simulink model "TeamA_PAsqualo1"  (R2020a)
settings: Solver=VariableStepAuto  StartTime=0.0  StopTime=stop_time  FixedStep=0.05  RelTol=1e-3
InitFcn:
  | main_init
values from neighbouring files (symbols this model uses):
  a1 = rho * D^4 * alpha1    (= 0.000388302366464)    [data_current.m]    (also in main_init.m)
  a2 = -rho * D^3 * alpha2 * (1 - omega)    (= 0.0037030698432)    [data_current.m]    (also in main_init.m)
  ag = [Ax Ay Az]'    [init_modello.m]
  alpha1 = 0.0113    [data_current.m]    (also in main_init.m)
  alpha2 = -0.0091    [data_current.m]    (also in main_init.m)
  areaOfInterestCorner = [42.317744;10.915136; 0]    [init_controllo.m]    (also in missionA.m = [42.317744)
  bg = [Bx By Bz]'    [init_modello.m]
  cd_pitch = 0.7    [init_modello.m]
  cd_roll = 0.04    [init_modello.m]
  cd_x = 0.4    [init_modello.m]
  cd_y = 1    [init_modello.m]
  cd_yaw = 0.7    [init_modello.m]
  cd_z = 1    [init_modello.m]
  cg = [Cx Cy Cz]'    [init_modello.m]
  D = 0.076    [data_current.m]    (also in main_init.m)
  dead_zone_limit = 31.5    [data_current.m]    (also in main_init.m)
  dg = [Dx Dy Dz]'    [init_modello.m]
  eg = [Ex Ey Ez]'    [init_modello.m]
  fg = [Fx Fy Fz]'    [init_modello.m]
  g = 9.81    [init_modello.m]
  galleggiamento = 66.5386    [init_controllo.m]
  gg = [Gx Gy Gz]'    [init_modello.m]
  H0 = 0    [init_modello.m]
  init_position = [pointP(1),pointP(2),0.15,0,0,deg2rad(angle)]'    [appunti.m]    (also in init_modello.m = [pointP(1),pointP(2),0.15,0,0,deg2rad(alpha)]')
  init_velocity = [0 0 0 0 0 0]'    [init_modello.m]
  initial_state_cov = blkdiag(diag(cov_gps(1,1:2)), cov_depth*eye(n_state_filter-2))    [init_navigazione.m]
  Ixx = 0.93304097392    [init_modello.m]
  Ixy = 0    [init_modello.m]
  Ixz = 0    [init_modello.m]
  Iyy = 25.58745481378    (= 25.5874548138)    [init_modello.m]
  Iyz = 0    [init_modello.m]
  Izz = 25.58745481378    (= 25.5874548138)    [init_modello.m]
  K_i_heave_div = 20    [init_controllo.m]
  K_i_heave_pos = 1    [init_controllo.m]
  K_i_heave_surf = 20    [init_controllo.m]
  K_i_heave_trans = 5    [init_controllo.m]
  K_i_heave_turn = 5    [init_controllo.m]
  K_i_pitch_div = 0    [init_controllo.m]
  K_i_pitch_pos = 0.1*0    (= 0)    [init_controllo.m]
  K_i_pitch_surf = 0    [init_controllo.m]
  K_i_pitch_trans = 0    [init_controllo.m]
  K_i_pitch_turn = 0    [init_controllo.m]
  K_i_roll_div = 0    [init_controllo.m]
  K_i_roll_pos = 0.1*0    (= 0)    [init_controllo.m]
  K_i_roll_surf = 1    [init_controllo.m]
  K_i_roll_trans = 0    [init_controllo.m]
  K_i_roll_turn = 0    [init_controllo.m]
  K_i_surge_div = 3    [init_controllo.m]
  K_i_surge_pos = 0.1679*30    (= 5.037)    [init_controllo.m]
  K_i_surge_surf = 3    [init_controllo.m]
  K_i_surge_trans = 0.1679*15    (= 2.5185)    [init_controllo.m]
  K_i_surge_turn = 0.1679*60    (= 10.074)    [init_controllo.m]
  K_i_sway_div = 6    [init_controllo.m]
  K_i_sway_pos = 5    [init_controllo.m]
  K_i_sway_surf = 3    [init_controllo.m]
  K_i_sway_trans = 2    [init_controllo.m]
  K_i_sway_turn = 50    [init_controllo.m]
  K_i_yaw_div = 0    [init_controllo.m]
  K_i_yaw_pos = 1    [init_controllo.m]
  K_i_yaw_surf = 0    [init_controllo.m]
  K_i_yaw_trans = 20    [init_controllo.m]
  K_i_yaw_turn = 3    [init_controllo.m]
  K_p_heave_div = 200    [init_controllo.m]
  K_p_heave_pos = 320    [init_controllo.m]
  K_p_heave_surf = 200    [init_controllo.m]
  K_p_heave_trans = 170    [init_controllo.m]
  K_p_heave_turn = 170    [init_controllo.m]
  K_p_phi_div = 0.15    [init_controllo.m]
  K_p_phi_pos = 1*0.1    (= 0.1)    [init_controllo.m]
  K_p_phi_surf = 0.15    [init_controllo.m]
  K_p_phi_trans = 0.1    [init_controllo.m]
  K_p_phi_turn = 0.1    [init_controllo.m]
  K_p_pitch_div = 50    [init_controllo.m]
  K_p_pitch_pos = 25    [init_controllo.m]
  K_p_pitch_surf = 50    [init_controllo.m]
  K_p_pitch_trans = 25    [init_controllo.m]
  K_p_pitch_turn = 25    [init_controllo.m]
  K_p_psi_div = 0.3    [init_controllo.m]
  K_p_psi_pos = 0.25    [init_controllo.m]
  K_p_psi_surf = 0.3    [init_controllo.m]
  K_p_psi_trans = 0.2    [init_controllo.m]
  K_p_roll_div = 10    [init_controllo.m]
  K_p_roll_pos = 0.1*40    (= 4)    [init_controllo.m]
  K_p_roll_surf = 10    [init_controllo.m]
  K_p_roll_trans = 0.1*40    (= 4)    [init_controllo.m]
  K_p_roll_turn = 4    [init_controllo.m]
  K_p_surge_div = 80    [init_controllo.m]
  K_p_surge_pos = 13.7782*2.5    (= 34.4455)    [init_controllo.m]
  K_p_surge_surf = 80    [init_controllo.m]
  K_p_surge_trans = 20    [init_controllo.m]
  K_p_surge_turn = 150    [init_controllo.m]
  K_p_sway_div = 100    [init_controllo.m]
  K_p_sway_pos = 90    [init_controllo.m]
  K_p_sway_surf = 80    [init_controllo.m]
  K_p_sway_trans = 80    [init_controllo.m]
  K_p_sway_turn = 200    [init_controllo.m]
  K_p_th_div = 0.3    [init_controllo.m]
  K_p_th_pos = 0.1    [init_controllo.m]
  K_p_th_surf = 0.3    [init_controllo.m]
  K_p_th_trans = 0.1    [init_controllo.m]
  K_p_th_turn = 0.1    [init_controllo.m]
  K_p_x_div = 0.12    [init_controllo.m]
  K_p_x_pos = 0.12    [init_controllo.m]
  K_p_x_surf = 0.12    [init_controllo.m]
  K_p_y_div = 0.6    [init_controllo.m]
  K_p_y_pos = 0.34    [init_controllo.m]
  K_p_y_surf = 0.1    [init_controllo.m]
  K_p_y_trans = 0.3    [init_controllo.m]
  K_p_y_turn = 0.3    [init_controllo.m]
  K_p_yaw_div = 70    [init_controllo.m]
  K_p_yaw_pos = 20    [init_controllo.m]
  K_p_yaw_surf = 70    [init_controllo.m]
  K_p_yaw_trans = 160    [init_controllo.m]
  K_p_yaw_turn = 60    [init_controllo.m]
  K_p_z_div = 0.35    [init_controllo.m]
  K_p_z_pos = 0.2    [init_controllo.m]
  K_p_z_surf = 0.35    [init_controllo.m]
  K_p_z_trans = 0.10    (= 0.1)    [init_controllo.m]
  K_p_z_turn = 0.1    [init_controllo.m]
  Kadd = 0    [init_modello.m]
  ... (+61 more)
undefined symbols (not defined in the file or in its folder): DiscIntNeverNeededParam, initial_state
libraries: simulink x4, vrlib x1
(part 3 of 6)

== system TeamA_PAsqualo1/Controller/surfacing controller/pitch_controller/Pitch PID controller ==
  enable : Inport
  references : Inport  Port=2
  "estimated measures " : Inport  Port=3
  Constant : Constant
  Constant1 : Constant  Value=0
  Discrete-Time Integrator : DiscreteIntegrator  ExternalReset=falling  SampleTime=0.1  ICPrevOutput=DiscIntNeverNeededParam  ICPrevScaledInput=DiscIntNeverNeededParam
  K_i_pitch_surf : Gain  Gain=K_i_pitch_surf
  K_p_pitch_surf : Gain  Gain=K_p_pitch_surf
  K_p_th_surf : Gain  Gain=K_p_th_surf
  Sum2 : Sum
  Switch : Switch  Threshold=1
  compute_orientation_errors : MATLAB Function  TreatAsAtomicUnit=on
  compute_velocity_error : MATLAB Function  TreatAsAtomicUnit=on
  M : Outport
  wires:
  references/1 -> compute_orientation_errors/2(ref)
  K_p_th_surf/1 -> compute_velocity_error/2(v_des)
  "estimated measures "/1 -> compute_velocity_error/3(est_meas), compute_orientation_errors/3(est_state)
  compute_orientation_errors/1(err_orient) -> K_p_th_surf/1  "err_orient"
  Sum2/1 -> M/1
  Discrete-Time Integrator/1 -> Sum2/2
  K_i_pitch_surf/1 -> Discrete-Time Integrator/1
  K_p_pitch_surf/1 -> Sum2/1
  compute_velocity_error/1(err_vel) -> K_i_pitch_surf/1, K_p_pitch_surf/1  "err_vel"
  Switch/1 -> Discrete-Time Integrator/2
  enable/1 -> Switch/2, compute_velocity_error/1(enable), compute_orientation_errors/1(enable)
  Constant1/1 -> Switch/3
  Constant/1 -> Switch/1

== system TeamA_PAsqualo1/Controller/surfacing controller/roll_controller/Roll PID controller ==
  enable : Inport
  references : Inport  Port=2
  "estimated measures " : Inport  Port=3
  Constant : Constant
  Constant1 : Constant  Value=0
  Discrete-Time Integrator : DiscreteIntegrator  ExternalReset=falling  SampleTime=0.1  ICPrevOutput=DiscIntNeverNeededParam  ICPrevScaledInput=DiscIntNeverNeededParam
  K_i_roll_surf : Gain  Gain=K_i_roll_surf
  K_p_phi_surf : Gain  Gain=K_p_phi_surf
  K_p_roll_surf : Gain  Gain=K_p_roll_surf
  Sum2 : Sum
  Switch : Switch  Threshold=1
  compute_orientation_errors : MATLAB Function  TreatAsAtomicUnit=on
  compute_velocity_error : MATLAB Function  TreatAsAtomicUnit=on
  K : Outport
  wires:
  "estimated measures "/1 -> compute_velocity_error/3(est_meas), compute_orientation_errors/3(est_state)
  K_p_phi_surf/1 -> compute_velocity_error/2(v_des)
  compute_orientation_errors/1(err_orient) -> K_p_phi_surf/1  "err_orient"
  references/1 -> compute_orientation_errors/2(ref)
  Sum2/1 -> K/1
  Discrete-Time Integrator/1 -> Sum2/2
  K_i_roll_surf/1 -> Discrete-Time Integrator/1
  K_p_roll_surf/1 -> Sum2/1
  compute_velocity_error/1(err_vel) -> K_i_roll_surf/1, K_p_roll_surf/1  "err_vel"
  Switch/1 -> Discrete-Time Integrator/2
  enable/1 -> Switch/2, compute_velocity_error/1(enable), compute_orientation_errors/1(enable)
  Constant1/1 -> Switch/3
  Constant/1 -> Switch/1

== system TeamA_PAsqualo1/Controller/surfacing controller/surge_controller/Surge PID controller ==
  enable : Inport
  references : Inport  Port=2
  "estimated measures " : Inport  Port=3
  Constant : Constant
  Constant1 : Constant  Value=0
  Discrete-Time Integrator : DiscreteIntegrator  ExternalReset=falling  SampleTime=0.1  ICPrevOutput=DiscIntNeverNeededParam  ICPrevScaledInput=DiscIntNeverNeededParam
  K_i_surge_surf : Gain  Gain=K_i_surge_surf
  K_p_surge_surf : Gain  Gain=K_p_surge_surf
  K_p_x_surf : Gain  Gain=K_p_x_surf
  Sum2 : Sum
  Switch : Switch  Threshold=1
  compute_position_errors : MATLAB Function  TreatAsAtomicUnit=on
  compute_velocity_error : MATLAB Function  TreatAsAtomicUnit=on
  X : Outport
  wires:
  references/1 -> compute_position_errors/2(ref)
  compute_position_errors/1(err_pos) -> K_p_x_surf/1  "err_vect"
  K_p_x_surf/1 -> compute_velocity_error/2(v_des)
  "estimated measures "/1 -> compute_velocity_error/3(est_meas), compute_position_errors/3(est_state)
  K_i_surge_surf/1 -> Discrete-Time Integrator/1
  K_p_surge_surf/1 -> Sum2/1
  Sum2/1 -> X/1
  compute_velocity_error/1(err_vel) -> K_i_surge_surf/1, K_p_surge_surf/1  "err_vel"
  Discrete-Time Integrator/1 -> Sum2/2
  Switch/1 -> Discrete-Time Integrator/2
  enable/1 -> Switch/2, compute_velocity_error/1(enable), compute_position_errors/1(enable)
  Constant1/1 -> Switch/3
  Constant/1 -> Switch/1

== system TeamA_PAsqualo1/Controller/surfacing controller/sway_controller/Sway PID controller ==
  enable : Inport
  references : Inport  Port=2
  "estimated measures " : Inport  Port=3
  Constant : Constant
  Constant1 : Constant  Value=0
  Discrete-Time Integrator : DiscreteIntegrator  ExternalReset=falling  SampleTime=0.1  ICPrevOutput=DiscIntNeverNeededParam  ICPrevScaledInput=DiscIntNeverNeededParam
  K_i_sway_surf : Gain  Gain=K_i_sway_surf
  K_p_sway_surf : Gain  Gain=K_p_sway_surf
  K_p_y_surf : Gain  Gain=K_p_y_surf
  Sum2 : Sum
  Switch : Switch  Threshold=1
  compute_position_errors : MATLAB Function  TreatAsAtomicUnit=on
  compute_velocity_error : MATLAB Function  TreatAsAtomicUnit=on
  Y : Outport
  wires:
  references/1 -> compute_position_errors/2(ref)
  compute_position_errors/1(err_pos) -> K_p_y_surf/1  "err_y"
  K_p_y_surf/1 -> compute_velocity_error/2(v_des)
  "estimated measures "/1 -> compute_velocity_error/3(est_meas), compute_position_errors/3(est_state)
  K_i_sway_surf/1 -> Discrete-Time Integrator/1
  K_p_sway_surf/1 -> Sum2/1
  Sum2/1 -> Y/1
  compute_velocity_error/1(err_vel) -> K_i_sway_surf/1, K_p_sway_surf/1  "err_vel"
  Discrete-Time Integrator/1 -> Sum2/2
  Switch/1 -> Discrete-Time Integrator/2
  enable/1 -> Switch/2, compute_velocity_error/1(enable), compute_position_errors/1(enable)
  Constant1/1 -> Switch/3
  Constant/1 -> Switch/1

== system TeamA_PAsqualo1/Controller/surfacing controller/yaw_controller/Yaw PID controller ==
  enable : Inport
  references : Inport  Port=2
  "estimated measures " : Inport  Port=3
  Constant : Constant
  Constant1 : Constant  Value=0
  Discrete-Time Integrator : DiscreteIntegrator  ExternalReset=falling  SampleTime=0.1  ICPrevOutput=DiscIntNeverNeededParam  ICPrevScaledInput=DiscIntNeverNeededParam
  K_i_yaw_surf : Gain  Gain=K_i_yaw_surf
  K_p_psi_surf : Gain  Gain=K_p_psi_surf
  K_p_yaw_surf : Gain  Gain=K_p_yaw_surf
  Sum2 : Sum
  Switch : Switch  Threshold=1
  compute_orientation_errors : MATLAB Function  TreatAsAtomicUnit=on
  compute_velocity_error : MATLAB Function  TreatAsAtomicUnit=on
  N : Outport
  wires:
  references/1 -> compute_orientation_errors/2(ref)
  "estimated measures "/1 -> compute_velocity_error/3(est_meas), compute_orientation_errors/3(est_state)
  compute_orientation_errors/1(err_orient) -> K_p_psi_surf/1  "err_orient"
  K_p_psi_surf/1 -> compute_velocity_error/2(v_des)
  Sum2/1 -> N/1
  Discrete-Time Integrator/1 -> Sum2/2
  K_i_yaw_surf/1 -> Discrete-Time Integrator/1
  K_p_yaw_surf/1 -> Sum2/1
  compute_velocity_error/1(err_vel) -> K_i_yaw_surf/1, K_p_yaw_surf/1  "err_vel"
  Switch/1 -> Discrete-Time Integrator/2
  enable/1 -> Switch/2, compute_velocity_error/1(enable), compute_orientation_errors/1(enable)
  Constant1/1 -> Switch/3
  Constant/1 -> Switch/1

== system TeamA_PAsqualo1/Controller/transect controller/heave_controller/Heave PID controller ==
  enable : Inport
  references : Inport  Port=2
  "estimated measures " : Inport  Port=3
  Constant : Constant  Value=galleggiamento
  Constant1 : Constant
  Constant2 : Constant  Value=0
  Discrete-Time Integrator : DiscreteIntegrator  ExternalReset=falling  InitialConditionSource=external  SampleTime=0.1  ICPrevOutput=DiscIntNeverNeededParam  ICPrevScaledInput=DiscIntNeverNeededParam
  K_i_heave_trans : Gain  Gain=K_i_heave_trans
  K_p_heave_trans : Gain  Gain=K_p_heave_trans
  K_p_z_trans : Gain  Gain=K_p_z_trans
  Sum2 : Sum
  Switch : Switch  Threshold=1
  compute_position_errors : MATLAB Function  TreatAsAtomicUnit=on
  compute_velocity_error : MATLAB Function  TreatAsAtomicUnit=on
  Z : Outport
  wires:
  "estimated measures "/1 -> compute_velocity_error/3(est_meas), compute_position_errors/3(est_state)
  K_p_z_trans/1 -> compute_velocity_error/2(v_des)
  compute_position_errors/1(err_pos) -> K_p_z_trans/1  "err_vect"
  references/1 -> compute_position_errors/2(ref)
  Sum2/1 -> Z/1
  Discrete-Time Integrator/1 -> Sum2/2
  K_p_heave_trans/1 -> Sum2/1
  K_i_heave_trans/1 -> Discrete-Time Integrator/1
  compute_velocity_error/1(err_vel) -> K_i_heave_trans/1, K_p_heave_trans/1  "err_vel"
  Constant/1 -> Discrete-Time Integrator/3
  Switch/1 -> Discrete-Time Integrator/2
  enable/1 -> Switch/2, compute_velocity_error/1(enable), compute_position_errors/1(enable)
  Constant2/1 -> Switch/3
  Constant1/1 -> Switch/1

== system TeamA_PAsqualo1/Controller/transect controller/pitch_controller/Pitch PID controller ==
  enable : Inport
  references : Inport  Port=2
  "estimated measures " : Inport  Port=3
  Constant : Constant
  Constant1 : Constant  Value=0
  Discrete-Time Integrator : DiscreteIntegrator  ExternalReset=falling  SampleTime=0.1  ICPrevOutput=DiscIntNeverNeededParam  ICPrevScaledInput=DiscIntNeverNeededParam
  K_i_pitch_trans : Gain  Gain=K_i_pitch_trans
  K_p_pitch_trans : Gain  Gain=K_p_pitch_trans
  K_p_th_trans : Gain  Gain=K_p_th_trans
  Sum2 : Sum
  Switch : Switch  Threshold=1
  compute_orientation_errors : MATLAB Function  TreatAsAtomicUnit=on
  compute_velocity_error : MATLAB Function  TreatAsAtomicUnit=on
  M : Outport
  wires:
  references/1 -> compute_orientation_errors/2(ref)
  K_p_th_trans/1 -> compute_velocity_error/2(v_des)
  "estimated measures "/1 -> compute_velocity_error/3(est_meas), compute_orientation_errors/3(est_state)
  compute_orientation_errors/1(err_orient) -> K_p_th_trans/1  "err_orient"
  Sum2/1 -> M/1
  Discrete-Time Integrator/1 -> Sum2/2
  K_p_pitch_trans/1 -> Sum2/1
  K_i_pitch_trans/1 -> Discrete-Time Integrator/1
  compute_velocity_error/1(err_vel) -> K_i_pitch_trans/1, K_p_pitch_trans/1  "err_vel"
  Switch/1 -> Discrete-Time Integrator/2
  enable/1 -> Switch/2, compute_velocity_error/1(enable), compute_orientation_errors/1(enable)
  Constant1/1 -> Switch/3
  Constant/1 -> Switch/1

== system TeamA_PAsqualo1/Controller/transect controller/roll_controller/Roll PID controller ==
  enable : Inport
  references : Inport  Port=2
  "estimated measures " : Inport  Port=3
  Constant : Constant
  Constant1 : Constant  Value=0
  Discrete-Time Integrator : DiscreteIntegrator  ExternalReset=falling  SampleTime=0.1  ICPrevOutput=DiscIntNeverNeededParam  ICPrevScaledInput=DiscIntNeverNeededParam
  K_i_roll_trans : Gain  Gain=K_i_roll_trans
  K_p_phi_trans : Gain  Gain=K_p_phi_trans
  K_p_roll_trans : Gain  Gain=K_p_roll_trans
  Sum2 : Sum
  Switch : Switch  Threshold=1
  compute_orientation_errors : MATLAB Function  TreatAsAtomicUnit=on
  compute_velocity_error : MATLAB Function  TreatAsAtomicUnit=on
  tau_roll : Outport
  wires:
  "estimated measures "/1 -> compute_velocity_error/3(est_meas), compute_orientation_errors/3(est_state)
  K_p_phi_trans/1 -> compute_velocity_error/2(v_des)
  compute_orientation_errors/1(err_orient) -> K_p_phi_trans/1  "err_orient"
  references/1 -> compute_orientation_errors/2(ref)
  Sum2/1 -> tau_roll/1
  Discrete-Time Integrator/1 -> Sum2/2
  K_p_roll_trans/1 -> Sum2/1
  K_i_roll_trans/1 -> Discrete-Time Integrator/1
  compute_velocity_error/1(err_vel) -> K_p_roll_trans/1, K_i_roll_trans/1  "err_vel"
  Switch/1 -> Discrete-Time Integrator/2
  Constant1/1 -> Switch/3
  Constant/1 -> Switch/1
  enable/1 -> Switch/2, compute_velocity_error/1(enable), compute_orientation_errors/1(enable)

== system TeamA_PAsqualo1/Controller/transect controller/surge_controller/Surge PID controller ==
  enable : Inport
  ref : Inport  Port=2
  est_meas : Inport  Port=3
  " compute_velocity_error" : MATLAB Function  TreatAsAtomicUnit=on
  Constant : Constant
  Constant1 : Constant  Value=0
  Discrete-Time Integrator : DiscreteIntegrator  ExternalReset=falling  SampleTime=0.1  ICPrevOutput=DiscIntNeverNeededParam  ICPrevScaledInput=DiscIntNeverNeededParam
  K_i_surge_trans : Gain  Gain=K_i_surge_trans
  K_p_surge_trans : Gain  Gain=K_p_surge_trans
  Scope : Scope
  Sum2 : Sum
  Switch : Switch  Threshold=1
  X : Outport
  wires:
  est_meas/1 -> " compute_velocity_error"/3(est_meas)
  ref/1 -> " compute_velocity_error"/2(ref)
  " compute_velocity_error"/1(err_vel) -> K_i_surge_trans/1, K_p_surge_trans/1  "err_vel"
  K_p_surge_trans/1 -> Sum2/1
  Sum2/1 -> Scope/1, X/1  "X"
  K_i_surge_trans/1 -> Discrete-Time Integrator/1
  Discrete-Time Integrator/1 -> Sum2/2
  Switch/1 -> Discrete-Time Integrator/2
  enable/1 -> Switch/2, " compute_velocity_error"/1(enable)
  Constant1/1 -> Switch/3
  Constant/1 -> Switch/1

== system TeamA_PAsqualo1/Controller/transect controller/sway_controller/Sway PID controller ==
  enable : Inport
  references : Inport  Port=2
  "estimated measures " : Inport  Port=3
  Constant : Constant
  Constant1 : Constant  Value=0
  Discrete-Time Integrator : DiscreteIntegrator  ExternalReset=falling  SampleTime=0.1  LimitOutput=on  ICPrevOutput=DiscIntNeverNeededParam  ICPrevScaledInput=DiscIntNeverNeededParam
  K_i_sway_trans : Gain  Gain=K_i_sway_trans
  K_p_sway_trans : Gain  Gain=K_p_sway_trans
  K_p_y_trans : Gain  Gain=K_p_y_trans
  Scope : Scope
  Sum2 : Sum
  Switch : Switch  Threshold=1
  compute_position_errors : MATLAB Function  TreatAsAtomicUnit=on
  compute_velocity_error : MATLAB Function  TreatAsAtomicUnit=on
  Y : Outport
  wires:
  references/1 -> compute_position_errors/2(ref)
  compute_position_errors/1(err_pos) -> K_p_y_trans/1  "err_vect"
  K_p_y_trans/1 -> compute_velocity_error/2(v_des)
  "estimated measures "/1 -> compute_velocity_error/3(est_meas), compute_position_errors/3(est_state)
  compute_velocity_error/1(err_vel) -> K_i_sway_trans/1, K_p_sway_trans/1  "err_vel"
  Discrete-Time Integrator/1 -> Scope/1, Sum2/2
  K_i_sway_trans/1 -> Discrete-Time Integrator/1
  Sum2/1 -> Y/1
  K_p_sway_trans/1 -> Sum2/1
  Switch/1 -> Discrete-Time Integrator/2
  enable/1 -> Switch/2, compute_velocity_error/1(enable), compute_position_errors/1(enable)
  Constant1/1 -> Switch/3
  Constant/1 -> Switch/1

== system TeamA_PAsqualo1/Controller/transect controller/yaw_controller/Yaw PID controller ==
  enable : Inport
  references : Inport  Port=2
  "estimated measures " : Inport  Port=3
  Constant : Constant
  Constant1 : Constant  Value=0
  Discrete-Time Integrator : DiscreteIntegrator  ExternalReset=falling  SampleTime=0.1  ICPrevOutput=DiscIntNeverNeededParam  ICPrevScaledInput=DiscIntNeverNeededParam
  K_i_yaw_trans : Gain  Gain=K_i_yaw_trans
  K_p_psi_trans : Gain  Gain=K_p_psi_trans
  K_p_yaw_trans : Gain  Gain=K_p_yaw_trans
  Sum2 : Sum
  Switch : Switch  Threshold=1
  compute_orientation_errors : MATLAB Function  TreatAsAtomicUnit=on
  compute_velocity_error : MATLAB Function  TreatAsAtomicUnit=on
  N : Outport
  wires:
  references/1 -> compute_orientation_errors/2(ref)
  "estimated measures "/1 -> compute_velocity_error/3(est_meas), compute_orientation_errors/3(est_state)
  compute_orientation_errors/1(err_orient) -> K_p_psi_trans/1  "err_orient"
  K_p_psi_trans/1 -> compute_velocity_error/2(v_des)
  Sum2/1 -> N/1
  Discrete-Time Integrator/1 -> Sum2/2
  K_p_yaw_trans/1 -> Sum2/1
  K_i_yaw_trans/1 -> Discrete-Time Integrator/1
  compute_velocity_error/1(err_vel) -> K_i_yaw_trans/1, K_p_yaw_trans/1  "err_vel"
  Switch/1 -> Discrete-Time Integrator/2
  enable/1 -> Switch/2, compute_velocity_error/1(enable), compute_orientation_errors/1(enable)
  Constant1/1 -> Switch/3
  Constant/1 -> Switch/1

== system TeamA_PAsqualo1/Controller/turning controller/heave_controller/Heave PID controller ==
  enable : Inport
  references : Inport  Port=2
  "estimated measures " : Inport  Port=3
  Constant : Constant  Value=galleggiamento
  Constant1 : Constant
  Constant2 : Constant  Value=0
  Discrete-Time Integrator : DiscreteIntegrator  ExternalReset=falling  InitialConditionSource=external  SampleTime=0.1  ICPrevOutput=DiscIntNeverNeededParam  ICPrevScaledInput=DiscIntNeverNeededParam
  K_i_heave_turn : Gain  Gain=K_i_heave_turn
  K_p_heave_turn : Gain  Gain=K_p_heave_turn
  K_p_z_turn : Gain  Gain=K_p_z_turn
  Sum2 : Sum
  Switch : Switch  Threshold=1
  compute_position_errors : MATLAB Function  TreatAsAtomicUnit=on
  compute_velocity_error : MATLAB Function  TreatAsAtomicUnit=on
  Z : Outport
  wires:
  "estimated measures "/1 -> compute_velocity_error/3(est_meas), compute_position_errors/3(est_state)
  K_p_z_turn/1 -> compute_velocity_error/2(v_des)
  compute_position_errors/1(err_pos) -> K_p_z_turn/1  "err_vect"
  references/1 -> compute_position_errors/2(ref)
  K_p_heave_turn/1 -> Sum2/1
  K_i_heave_turn/1 -> Discrete-Time Integrator/1
  Discrete-Time Integrator/1 -> Sum2/2
  Sum2/1 -> Z/1
  compute_velocity_error/1(err_vel) -> K_i_heave_turn/1, K_p_heave_turn/1  "err_vel"
  Constant/1 -> Discrete-Time Integrator/3
  Switch/1 -> Discrete-Time Integrator/2
  enable/1 -> Switch/2, compute_velocity_error/1(enable), compute_position_errors/1(enable)
  Constant2/1 -> Switch/3
  Constant1/1 -> Switch/1

== system TeamA_PAsqualo1/Controller/turning controller/pitch_controller/Pitch PID controller ==
  enable : Inport
  references : Inport  Port=2
  "estimated measures " : Inport  Port=3
  Constant : Constant
  Constant1 : Constant  Value=0
  Discrete-Time Integrator : DiscreteIntegrator  ExternalReset=falling  SampleTime=0.1  ICPrevOutput=DiscIntNeverNeededParam  ICPrevScaledInput=DiscIntNeverNeededParam
  K_i_pitch_turn : Gain  Gain=K_i_pitch_turn
  K_p_pitch_turn : Gain  Gain=K_p_pitch_turn
  K_p_th_turn : Gain  Gain=K_p_th_turn
  Sum2 : Sum
  Switch : Switch  Threshold=1
  compute_orientation_errors : MATLAB Function  TreatAsAtomicUnit=on
  compute_velocity_error : MATLAB Function  TreatAsAtomicUnit=on
  M : Outport
  wires:
  references/1 -> compute_orientation_errors/2(ref)
  K_p_th_turn/1 -> compute_velocity_error/2(v_des)
  "estimated measures "/1 -> compute_velocity_error/3(est_meas), compute_orientation_errors/3(est_state)
  compute_orientation_errors/1(err_orient) -> K_p_th_turn/1  "err_orient"
  Sum2/1 -> M/1
  compute_velocity_error/1(err_vel) -> K_i_pitch_turn/1, K_p_pitch_turn/1  "err_vel"
  Discrete-Time Integrator/1 -> Sum2/2
  K_p_pitch_turn/1 -> Sum2/1
  K_i_pitch_turn/1 -> Discrete-Time Integrator/1
  Switch/1 -> Discrete-Time Integrator/2
  enable/1 -> Switch/2, compute_velocity_error/1(enable), compute_orientation_errors/1(enable)
  Constant1/1 -> Switch/3
  Constant/1 -> Switch/1

== system TeamA_PAsqualo1/Controller/turning controller/roll_controller/Roll PID controller ==
  enable : Inport
  references : Inport  Port=2
  "estimated measures " : Inport  Port=3
  Constant : Constant
  Constant1 : Constant  Value=0
  Discrete-Time Integrator : DiscreteIntegrator  ExternalReset=falling  SampleTime=0.1  ICPrevOutput=DiscIntNeverNeededParam  ICPrevScaledInput=DiscIntNeverNeededParam
  K_i_roll_turn : Gain  Gain=K_i_roll_turn
  K_p_phi_turn : Gain  Gain=K_p_phi_turn
  K_p_roll_turn : Gain  Gain=K_p_roll_turn
  Sum2 : Sum
  Switch : Switch  Threshold=1
  compute_orientation_errors : MATLAB Function  TreatAsAtomicUnit=on
  compute_velocity_error : MATLAB Function  TreatAsAtomicUnit=on
  K : Outport
  wires:
  "estimated measures "/1 -> compute_velocity_error/3(est_meas), compute_orientation_errors/3(est_state)
  K_p_phi_turn/1 -> compute_velocity_error/2(v_des)
  compute_orientation_errors/1(err_orient) -> K_p_phi_turn/1  "err_orient"
  references/1 -> compute_orientation_errors/2(ref)
  Sum2/1 -> K/1
  compute_velocity_error/1(err_vel) -> K_i_roll_turn/1, K_p_roll_turn/1  "err_vel"
  Discrete-Time Integrator/1 -> Sum2/2
  K_p_roll_turn/1 -> Sum2/1
  K_i_roll_turn/1 -> Discrete-Time Integrator/1
  Switch/1 -> Discrete-Time Integrator/2
  enable/1 -> Switch/2, compute_velocity_error/1(enable), compute_orientation_errors/1(enable)
  Constant1/1 -> Switch/3
  Constant/1 -> Switch/1

== system TeamA_PAsqualo1/Controller/turning controller/surge_controller/Surge PID controller ==
  enable : Inport
  ref : Inport  Port=2
  est_meas : Inport  Port=3
  " compute_velocity_error" : MATLAB Function  TreatAsAtomicUnit=on
  Constant : Constant
  Constant1 : Constant  Value=0
  Constant2 : Constant  Value=turning_surge
  Discrete-Time Integrator : DiscreteIntegrator  ExternalReset=falling  InitialConditionSource=external  SampleTime=0.1  ICPrevOutput=DiscIntNeverNeededParam  ICPrevScaledInput=DiscIntNeverNeededParam
  K_i_surge_turn : Gain  Gain=K_i_surge_turn
  K_p_surge_turn : Gain  Gain=K_p_surge_turn
  Scope : Scope
  Sum2 : Sum
  Switch : Switch  Threshold=1
  X : Outport
  wires:
  est_meas/1 -> " compute_velocity_error"/3(est_meas)
  ref/1 -> " compute_velocity_error"/2(ref)
  Sum2/1 -> Scope/1, X/1
  Discrete-Time Integrator/1 -> Sum2/2
  K_p_surge_turn/1 -> Sum2/1
  K_i_surge_turn/1 -> Discrete-Time Integrator/1
  " compute_velocity_error"/1(err_vel) -> K_i_surge_turn/1, K_p_surge_turn/1  "err_vel"
  Switch/1 -> Discrete-Time Integrator/2
  enable/1 -> Switch/2, " compute_velocity_error"/1(enable)
  Constant1/1 -> Switch/3
  Constant/1 -> Switch/1
  Constant2/1 -> Discrete-Time Integrator/3

== system TeamA_PAsqualo1/Controller/turning controller/sway_controller/Sway PID controller ==
  enable : Inport
  references : Inport  Port=2
  "estimated measures " : Inport  Port=3
  Constant : Constant
  Constant1 : Constant  Value=0
  Discrete-Time Integrator : DiscreteIntegrator  ExternalReset=falling  SampleTime=0.1  ICPrevOutput=DiscIntNeverNeededParam  ICPrevScaledInput=DiscIntNeverNeededParam
  K_i_sway_turn : Gain  Gain=K_i_sway_turn
  K_p_sway_turn : Gain  Gain=K_p_sway_turn
  K_p_y_turn : Gain  Gain=K_p_y_turn
  Scope : Scope
  Sum2 : Sum
  Switch : Switch  Threshold=1
  compute_position_errors : MATLAB Function  TreatAsAtomicUnit=on
  compute_velocity_error : MATLAB Function  TreatAsAtomicUnit=on
  Y : Outport
  wires:
  references/1 -> compute_position_errors/2(ref)
  compute_position_errors/1(err_pos) -> K_p_y_turn/1  "err_vect"
  K_p_y_turn/1 -> compute_velocity_error/2(v_des)
  "estimated measures "/1 -> compute_velocity_error/3(est_meas), compute_position_errors/3(est_state)
  K_p_sway_turn/1 -> Sum2/1
  K_i_sway_turn/1 -> Discrete-Time Integrator/1
  Discrete-Time Integrator/1 -> Scope/1, Sum2/2
  compute_velocity_error/1(err_vel) -> K_i_sway_turn/1, K_p_sway_turn/1  "err_vel"
  Sum2/1 -> Y/1
  Switch/1 -> Discrete-Time Integrator/2
  enable/1 -> Switch/2, compute_velocity_error/1(enable), compute_position_errors/1(enable)
  Constant1/1 -> Switch/3
  Constant/1 -> Switch/1

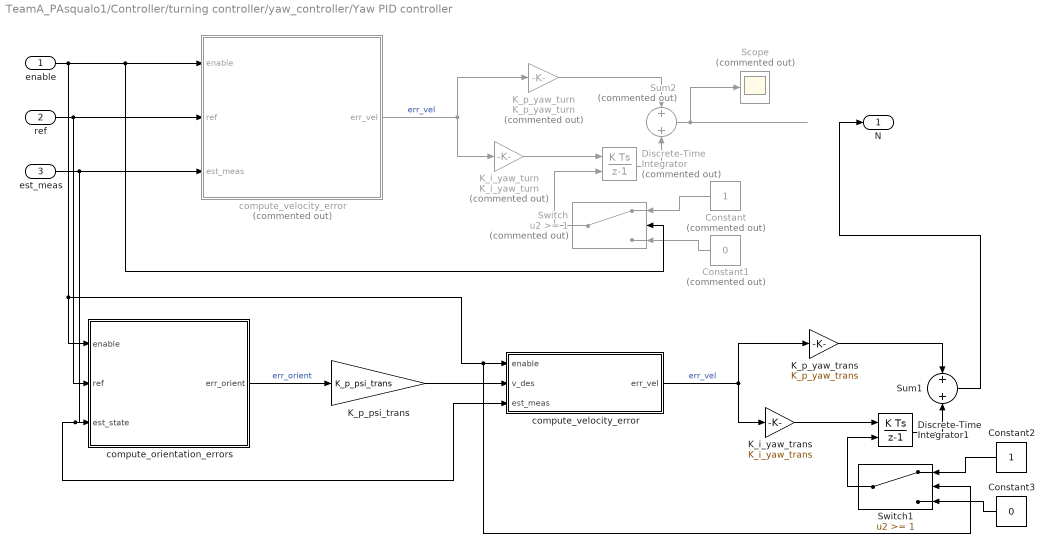
== system TeamA_PAsqualo1/Controller/turning controller/yaw_controller/Yaw PID controller ==
  enable : Inport
  ref : Inport  Port=2
  est_meas : Inport  Port=3
  " compute_velocity_error" : MATLAB Function  Commented=on  TreatAsAtomicUnit=on
  Constant : Constant  Commented=on
  Constant1 : Constant  Commented=on  Value=0
  Constant2 : Constant
  Constant3 : Constant  Value=0
  Discrete-Time Integrator : DiscreteIntegrator  Commented=on  ExternalReset=falling  SampleTime=0.1  ICPrevOutput=DiscIntNeverNeededParam  ICPrevScaledInput=DiscIntNeverNeededParam
  Discrete-Time Integrator1 : DiscreteIntegrator  ExternalReset=falling  SampleTime=0.1  ICPrevOutput=DiscIntNeverNeededParam  ICPrevScaledInput=DiscIntNeverNeededParam
  K_i_yaw_trans : Gain  Gain=K_i_yaw_trans
  K_i_yaw_turn : Gain  Commented=on  Gain=K_i_yaw_turn
  K_p_psi_trans : Gain  Gain=K_p_psi_trans
  K_p_yaw_trans : Gain  Gain=K_p_yaw_trans
  K_p_yaw_turn : Gain  Commented=on  Gain=K_p_yaw_turn
  Scope : Scope  Commented=on
  Sum1 : Sum
  Sum2 : Sum  Commented=on
  Switch : Switch  Commented=on  Threshold=1
  Switch1 : Switch  Threshold=1
  compute_orientation_errors : MATLAB Function  TreatAsAtomicUnit=on
  compute_velocity_error : MATLAB Function  TreatAsAtomicUnit=on
  N : Outport
  wires:
  Sum2/1 -> Scope/1
  " compute_velocity_error"/1(err_vel) -> K_i_yaw_turn/1, K_p_yaw_turn/1  "err_vel"
  Discrete-Time Integrator/1 -> Sum2/2
  K_p_yaw_turn/1 -> Sum2/1
  K_i_yaw_turn/1 -> Discrete-Time Integrator/1
  Switch/1 -> Discrete-Time Integrator/2
  Constant1/1 -> Switch/3
  Constant/1 -> Switch/1
  Constant3/1 -> Switch1/3
  Constant2/1 -> Switch1/1
  K_p_psi_trans/1 -> compute_velocity_error/2(v_des)
  Switch1/1 -> Discrete-Time Integrator1/2
  compute_velocity_error/1(err_vel) -> K_i_yaw_trans/1, K_p_yaw_trans/1  "err_vel"
  enable/1 -> compute_orientation_errors/1(enable), Switch1/2, compute_velocity_error/1(enable), Switch/2, " compute_velocity_error"/1(enable)
  K_i_yaw_trans/1 -> Discrete-Time Integrator1/1
  compute_orientation_errors/1(err_orient) -> K_p_psi_trans/1  "err_orient"
  est_meas/1 -> " compute_velocity_error"/3(est_meas), compute_velocity_error/3(est_meas), compute_orientation_errors/3(est_state)
  K_p_yaw_trans/1 -> Sum1/1
  ref/1 -> compute_orientation_errors/2(ref), " compute_velocity_error"/2(ref)
  Discrete-Time Integrator1/1 -> Sum1/2
  Sum1/1 -> N/1

== system TeamA_PAsqualo1/Navigazione/Selettore Misure/Selettore misure/pulse ==
  in : Inport
  Delay : Delay  DelayLength=1  SampleTime=ts_filter
  MATLAB Function : MATLAB Function  TreatAsAtomicUnit=on
  Scope : Scope
  Scope1 : Scope
  Sum2 : Sum  Inputs=|+-
  pulse : Outport
  wires:
  Sum2/1 -> MATLAB Function/2(u)
  in/1 -> Scope1/1, Delay/1, Sum2/1, MATLAB Function/1(gps_now)
  Delay/1 -> Sum2/2
  MATLAB Function/1(y) -> Scope/1, pulse/1

== system TeamA_PAsqualo1/Navigazione/Selettore Misure/Selettore misure/pulse2 ==
  in : Inport
  Delay : Delay  DelayLength=1  SampleTime=ts_filter
  MATLAB Function : MATLAB Function  TreatAsAtomicUnit=on
  Sum2 : Sum  Inputs=|+-
  pulse : Outport
  wires:
  Sum2/1 -> MATLAB Function/1(u)
  in/1 -> Delay/1, Sum2/1
  Delay/1 -> Sum2/2
  MATLAB Function/1(y) -> pulse/1

== system TeamA_PAsqualo1/Navigazione/Selettore Misure/Selettore misure/pulse4 ==
  in : Inport
  Delay : Delay  DelayLength=1  SampleTime=ts_filter
  MATLAB Function : MATLAB Function  TreatAsAtomicUnit=on
  Sum2 : Sum  Inputs=|+-
  pulse : Outport
  wires:
  Sum2/1 -> MATLAB Function/1(u)
  in/1 -> Delay/1, Sum2/1
  Delay/1 -> Sum2/2
  MATLAB Function/1(y) -> pulse/1

== matlab function TeamA_PAsqualo1/Vehicle Model/Damping computation ==
  data: nir input; D_effect output double size=[6 1]; cd_x parameter; cd_y parameter; cd_z parameter; cd_roll parameter; cd_pitch parameter; cd_yaw parameter; S_x parameter; S_y parameter; S_z parameter; S_roll parameter; S_pitch parameter; r_mz parameter; r_my parameter; r_mx parameter; S_yaw parameter; rho parameter
function D_effect = fcn(nir, cd_x, cd_y, cd_z, cd_roll, cd_pitch, cd_yaw, S_x, S_y, S_z, S_roll, S_pitch, r_mz, r_my, r_mx, S_yaw, rho)
%Calcolo matrice di Damping

vx = abs(nir(1));
vy = abs(nir(2));
vz = abs(nir(3));
wr = abs(nir(4));
wp = abs(nir(5));
wy = abs(nir(6));

D_x = -(1/2)*rho*cd_x*S_x*vx; %kg/m^3 * m^2 * m/s = kg/s (*m/s = N)
D_y = -(1/2)*rho*cd_y*S_y*vy;
D_z = -(1/2)*rho*cd_z*S_z*vz;

D_r = -(1/2)*rho*cd_roll*S_roll*((r_mx)^3)*wr; %kg/m^3 * m^2 * m^3 * 1/s = kg*m^2/s (*1/s = Nm)
D_p = -(1/2)*rho*cd_pitch*S_pitch*((r_my)^3)*wp;
D_yaw = -(1/2)*rho*cd_yaw*S_yaw*((r_mz)^3)*wy;

D = -blkdiag(D_x,D_y,D_z,D_r,D_p,D_yaw);

D_effect = D*nir;
end

== matlab function TeamA_PAsqualo1/Vehicle Model/Gravity computation ==
  data: g_effect output double size=[6 1]; J1 input double size=[3 3]; Rb parameter; Rg parameter; W parameter; eta input; V parameter; rho parameter; g parameter
function g_effect = fcn(J1, Rb, Rg, W, eta,V, rho, g)
B = V*rho*g*[0 0 -1]'; %Forza galleggiamento in terna NED
J1_inv = inv(J1);
Fw = J1_inv*W; %Peso in terna Body
if eta(3) < -0.15
    Fb = [0,0,0]';
else
    if eta(3) <= 0.15
        B = ((eta(3)+0.15)/0.3)*B;
        Fb = J1_inv*B; %Galleggiamento in terna Body
    else
        Fb = J1_inv*B; %Galleggiamento in terna Body
    end
end
g_effect = -[Fw+Fb;cross(Rg,Fw)+cross(Rb,Fb)];
end

== matlab function TeamA_PAsqualo1/Vehicle Model/Thruster E/MATLAB Function ==
  data: n input; T output; V input; D parameter; omega parameter; a1 parameter; a2 parameter; alpha1 parameter; alpha2 parameter
function T = thrusterModel(n, V, D, omega, a1, a2, alpha1, alpha2)

Va = (1-omega) * V;     % Advancement velocity at the propeller
J0 = Va/(n*D);          % Advancement Coefficient

if J0 > -alpha1/alpha2  % Out of linearity domain (right side)
    T = 0;              % A null generated thrust is assumed
    
elseif J0 < 0           % Out of linearity domain (left side)
    T = a1*abs(n)*n;    % Bollard thrust is assumed

else                    % Within the linearity domain
    T = a1*abs(n)*n - a2*abs(n)*V;
end

== matlab function TeamA_PAsqualo1/Vehicle Model/Thruster F/MATLAB Function ==
  data: n input; T output; V input; D parameter; omega parameter; a1 parameter; a2 parameter; alpha1 parameter; alpha2 parameter
function T = thrusterModel(n, V, D, omega, a1, a2, alpha1, alpha2)

Va = (1-omega) * V;     % Advancement velocity at the propeller
J0 = Va/(n*D);          % Advancement Coefficient

if J0 > -alpha1/alpha2  % Out of linearity domain (right side)
    T = 0;              % A null generated thrust is assumed
    
elseif J0 < 0           % Out of linearity domain (left side)
    T = a1*abs(n)*n;    % Bollard thrust is assumed

else                    % Within the linearity domain
    T = a1*abs(n)*n - a2*abs(n)*V;
end

== matlab function TeamA_PAsqualo1/Vehicle Model/MATLAB Function1 ==
  data: nir input double size=[6 1]; J1 input double size=[3 3]; ni_abs output double size=[6 1]; current_speed parameter double size=[3 1]
function ni_abs= fcn(nir,J1,current_speed)
J1_inv = inv(J1);
current_speed_Body = J1_inv*current_speed; %NED to Body computation
nir1 = [nir(1) nir(2) nir(3)]';
ni1_abs = nir1+current_speed_Body;
ni_abs = [ni1_abs(1) ni1_abs(2) ni1_abs(3) nir(4) nir(5) nir(6)]';
end

== matlab function TeamA_PAsqualo1/Vehicle Model/J computation ==
  data: J output double size=[6 6]; eta input double size=[6 1]
function J  = fcn(eta)
phi = eta(4);
theta = eta(5);
psi = eta(6);
Rx = [1 0 0;0 cos(phi) sin(phi);0 -sin(phi) cos(phi)];
Ry = [cos(theta) 0 -sin(theta);0 1 0;sin(theta) 0 cos(theta)];
Rz = [cos(psi) sin(psi) 0;-sin(psi) cos(psi) 0; 0 0 1];
J1 = Rz'*Ry'*Rx';
J2_inv = [1 0 -sin(theta);0 cos(phi) (cos(theta)*sin(phi));0 -sin(phi) (cos(theta)*cos(phi))];
J2 = inv(J2_inv);
J = [J1 zeros(3);zeros(3) J2];
end

== matlab function TeamA_PAsqualo1/Vehicle Model/MATLAB Function2 ==
  data: eta input double size=[6 1]; orient_true output
function orient_true = fcn(eta)
coder.extrinsic('wrapToPi');
orient_true = [0; 0; 0];
rr = eta(4);
r = wrapToPi(rr); %phi
pp = eta(5);
p = wrapToPi(pp); %theta
yy = eta(6);
y = wrapToPi(yy); %psi
orient_true = [r p y]';
end

== matlab function TeamA_PAsqualo1/Vehicle Model/MATLAB Function3 ==
  data: ni_abs input double size=[6 1]; vel_true output double size=[3 1]
function vel_true = fcn(ni_abs)
vx = ni_abs(1);
vy = ni_abs(2);
vz = ni_abs(3);
vel_true = [vx,vy,vz]';
end

== matlab function TeamA_PAsqualo1/Vehicle Model/MATLAB Function4 ==
  data: ni_abs input double size=[6 1]; w_true output double size=[3 1]
function w_true = fcn(ni_abs)
w_x = ni_abs(4);
w_y = ni_abs(5);
w_z = ni_abs(6);
w_true = [w_x,w_y,w_z]';
end

== matlab function TeamA_PAsqualo1/Vehicle Model/Thruster G/MATLAB Function ==
  data: n input; T output; V input; D parameter; omega parameter; a1 parameter; a2 parameter; alpha1 parameter; alpha2 parameter
function T = thrusterModel(n, V, D, omega, a1, a2, alpha1, alpha2)

Va = (1-omega) * V;     % Advancement velocity at the propeller
J0 = Va/(n*D);          % Advancement Coefficient

if J0 > -alpha1/alpha2  % Out of linearity domain (right side)
    T = 0;              % A null generated thrust is assumed
    
elseif J0 < 0           % Out of linearity domain (left side)
    T = a1*abs(n)*n;    % Bollard thrust is assumed

else                    % Within the linearity domain
    T = a1*abs(n)*n - a2*abs(n)*V;
end

== matlab function TeamA_PAsqualo1/Vehicle Model/Velocità_ai_thruster ==
  data: nir input double size=[6 1]; Va_rel output; Vb_rel output; Vc_rel output; Vd_rel output; Ve_rel output; Vf_rel output; Vg_rel output; orA parameter; orB parameter; orC parameter; orD parameter; orE parameter; orF parameter; orG parameter; ag parameter; bg parameter; cg parameter; dg parameter; eg parameter; fg parameter; gg parameter
function [Va_rel,Vb_rel,Vc_rel,Vd_rel,Ve_rel,Vf_rel,Vg_rel] = fcn(nir, orA, orB, orC, orD, orE, orF, orG, ag, bg, cg, dg, eg, fg, gg)
nir1 = [nir(1) nir(2) nir(3)]';
nir2 = [nir(4) nir(5) nir(6)]';
%Vettori orientazione thrusterX denominati orX  disponibili nel file init
%Vettori posizione thrusterX denominati xg disponibili nel file init
Va_rel = orA*(nir1 + cross(nir2,ag));
Vb_rel = orB*(nir1 + cross(nir2,bg));
Vc_rel = orC*(nir1 + cross(nir2,cg));
Vd_rel = orD*(nir1 + cross(nir2,dg));
Ve_rel = orE*(nir1 + cross(nir2,eg));
Vf_rel = orF*(nir1 + cross(nir2,fg));
Vg_rel = orG*(nir1 + cross(nir2,gg));
[Va_rel,Vb_rel,Vc_rel,Vd_rel,Ve_rel,Vf_rel,Vg_rel];
end

== matlab function TeamA_PAsqualo1/Vehicle Model/J1 computation ==
  data: eta input; J1 output
function J1 = fcn(eta)
phi = eta(4);
theta = eta(5);
psi = eta(6);
Rx = [1 0 0;0 cos(phi) sin(phi);0 -sin(phi) cos(phi)];
Ry = [cos(theta) 0 -sin(theta);0 1 0;sin(theta) 0 cos(theta)];
Rz = [cos(psi) sin(psi) 0;-sin(psi) cos(psi) 0; 0 0 1];
J1 = Rz'*Ry'*Rx';
end

== matlab function TeamA_PAsqualo1/Vehicle Model/ni_dot computation ==
  data: M_times_nir_dot input double size=[6 1]; nir_dot output double size=[6 1]; M_inv parameter
function nir_dot = fcn(M_times_nir_dot, M_inv)
nir_dot = M_inv * M_times_nir_dot;
end

== matlab function TeamA_PAsqualo1/Vehicle Model/ni_to_eta_dot ==
  data: J input; ni_abs input; eta_dot output
function eta_dot = fcn(J,ni_abs)
eta_dot = J*ni_abs;
end

== matlab function TeamA_PAsqualo1/Sensors and Environment Models /Global Positioning System/WGS84toNed  ==
  data: posizione input; posizione_NED output
function posizione_NED = wgs84toNed(posizione)

coder.extrinsic('evalin', 'wgs84Ellipsoid', 'geodetic2ned');
NED_origin = [0;0;0];
posizione_NED  = [0;0;0];
NED_origin = evalin('base', 'NED_origin');
[a, b, c] = geodetic2ned(posizione(1), posizione(2), posizione(3), NED_origin(1), NED_origin(2), NED_origin(3), wgs84Ellipsoid);
posizione_NED = [a; b; posizione(3)];

end

== matlab function TeamA_PAsqualo1/Sensors and Environment Models /Profondimetro/WGS84toNed  ==
  data: posizione input; posizione_NED output
function posizione_NED = wgs84toNed(posizione)

coder.extrinsic('evalin', 'wgs84Ellipsoid', 'geodetic2ned');
NED_origin = [0;0;0];
posizione_NED  = [0;0;0];
NED_origin = evalin('base', 'NED_origin');
[a, b, c] = geodetic2ned(posizione(1), posizione(2), posizione(3), NED_origin(1), NED_origin(2), NED_origin(3), wgs84Ellipsoid);
posizione_NED = [a; b; posizione(3)];

end

== matlab function TeamA_PAsqualo1/Sensors and Environment Models /Sonar_down/MATLAB Function ==
  data: posizione input; p_sonar_ned output; orientazione input; s_versor_ned output; tilt input; p_sonar_body input
function [p_sonar_ned, s_versor_ned] = rot_body_ned(posizione,orientazione,tilt,p_sonar_body)
   
 roll = orientazione(1);
 pitch = orientazione(2);
 yaw = orientazione(3);
 xNorth = posizione(1);
 yEast = posizione(2);
 zDown = posizione(3);
 Rx = [1 0 0; 0 cos(roll) -sin(roll); 0 sin(roll) cos(roll)];
 Ry = [cos(pitch) 0 sin(pitch); 0 1 0; -sin(pitch) 0 cos(pitch)];
 Rz = [cos(yaw) -sin(yaw) 0; sin(yaw) cos(yaw) 0; 0 0 1];
 J1 = Rz*Ry*Rx; %matrice di rotazione da body a ned frame 

 s_versor_body = [sin(tilt); 0 ; cos(tilt)];	% direzione sonar in terna body
 s_versor_ned = J1*s_versor_body;
 
 cs2sensor_ned = J1*p_sonar_body; % distanza cds-sensore in Ned
 %Posizione sensore in Ned frame:
 p_sonar_ned = [xNorth; yEast; zDown] + cs2sensor_ned;
end

== matlab function TeamA_PAsqualo1/Sensors and Environment Models /Sonar_down/MATLAB Function1 ==
  data: p_sonar_ned input; sol_t output; s_versor_ned input
function sol_t = sonar_down(p_sonar_ned, s_versor_ned)

coder.extrinsic('seabed_function');
sol_t = 0;
sol_t = seabed_function(p_sonar_ned, s_versor_ned);

end

== matlab function TeamA_PAsqualo1/Sensors and Environment Models /Sonar_down/WGS84toNed 1 ==
  data: posizione input; posizione_NED output
function posizione_NED = wgs84toNed(posizione)

coder.extrinsic('evalin', 'wgs84Ellipsoid', 'geodetic2ned');
NED_origin = [0;0;0];
posizione_NED  = [0;0;0];
NED_origin = evalin('base', 'NED_origin');
[a, b, c] = geodetic2ned(posizione(1), posizione(2), posizione(3), NED_origin(1), NED_origin(2), NED_origin(3), wgs84Ellipsoid);
posizione_NED = [a; b; posizione(3)];

end

== matlab function TeamA_PAsqualo1/Sensors and Environment Models /Sonar_front/MATLAB Function ==
  data: posizione input; p_sonar_ned output; orientazione input; s_versor_ned output; tilt input; p_sonar_body input
function [p_sonar_ned, s_versor_ned] = rot_body_ned(posizione,orientazione,tilt,p_sonar_body)
   
 roll = orientazione(1);
 pitch = orientazione(2);
 yaw = orientazione(3);
 xNorth = posizione(1);
 yEast = posizione(2);
 zDown = posizione(3);
 Rx = [1 0 0; 0 cos(roll) -sin(roll); 0 sin(roll) cos(roll)];
 Ry = [cos(pitch) 0 sin(pitch); 0 1 0; -sin(pitch) 0 cos(pitch)];
 Rz = [cos(yaw) -sin(yaw) 0; sin(yaw) cos(yaw) 0; 0 0 1];
 J1 = Rz*Ry*Rx; %matrice di rotazione da body a ned frame 

 s_versor_body = [sin(tilt); 0 ; cos(tilt)];	% direzione sonar in terna body
 s_versor_ned = J1*s_versor_body;
 
 cs2sensor_ned = J1*p_sonar_body; % distanza cds-sensore in Ned
 %Posizione sensore in Ned frame:
 p_sonar_ned = [xNorth; yEast; zDown] + cs2sensor_ned;
end

== matlab function TeamA_PAsqualo1/Sensors and Environment Models /Sonar_front/MATLAB Function1 ==
  data: p_sonar_ned input; sol_t output; s_versor_ned input
function sol_t = sonar_down(p_sonar_ned, s_versor_ned)

coder.extrinsic('seabed_function');
sol_t = 0;
sol_t = seabed_function(p_sonar_ned, s_versor_ned);

end

== matlab function TeamA_PAsqualo1/Sensors and Environment Models /Sonar_front/WGS84toNed 1 ==
  data: posizione input; posizione_NED output
function posizione_NED = wgs84toNed(posizione)

coder.extrinsic('evalin', 'wgs84Ellipsoid', 'geodetic2ned');
NED_origin = [0;0;0];
posizione_NED  = [0;0;0];
NED_origin = evalin('base', 'NED_origin');
[a, b, c] = geodetic2ned(posizione(1), posizione(2), posizione(3), NED_origin(1), NED_origin(2), NED_origin(3), wgs84Ellipsoid);
posizione_NED = [a; b; posizione(3)];

end

== matlab function TeamA_PAsqualo1/Sensors and Environment Models /Ultra Short Base Line System/MATLAB Function1 ==
  data: x_t_usbl input; bearing output; y_t_usbl input; z_t_usbl input; elevation output; range output
function [bearing,elevation,range] = usbl(x_t_usbl, y_t_usbl, z_t_usbl)
%coordinate sferiche in uscita dal sensore
range = sqrt((x_t_usbl)^2+(y_t_usbl)^2+(z_t_usbl^2)); 
elevation = asin(z_t_usbl/range);
bearing = atan2(y_t_usbl,x_t_usbl); 

 end

== matlab function TeamA_PAsqualo1/Sensors and Environment Models /Ultra Short Base Line System/MATLAB Function2 ==
  data: posizione input; x_t_usbl output; orientazione input; p_usbl input; p_transponder input; y_t_usbl output; z_t_usbl output
function [x_t_usbl,y_t_usbl,z_t_usbl]= rot_ned_usbl(posizione,orientazione, p_usbl, p_transponder)
 
roll = orientazione(1);
pitch = orientazione(2);
yaw = orientazione(3);
xNorth = posizione(1);
yEast = posizione(2);
zDown = posizione(3);
Rx = [1 0 0; 0 cos(roll) -sin(roll); 0 sin(roll) cos(roll)];
Ry = [cos(pitch) 0 sin(pitch); 0 1 0; -sin(pitch) 0 cos(pitch)];
Rz = [cos(yaw) -sin(yaw) 0; sin(yaw) cos(yaw) 0; 0 0 1];
J1 = Rz*Ry*Rx; %matrice di rotazione da body a ned frame 
p_usbl_ned = J1*p_usbl; % offset sensore -centro di simmetria riportato in terna ned 
p_sensore = p_usbl_ned + [xNorth;yEast;zDown]; %posizione sensore in
% terna ned 
b2transp_ned = p_transponder - p_sensore; %distanza trasponder-usbl in terna ned 
x_t_usbl = b2transp_ned(1);
y_t_usbl = b2transp_ned(2);
z_t_usbl = b2transp_ned(3);

end

== matlab function TeamA_PAsqualo1/Sensors and Environment Models /Ultra Short Base Line System/WGS84toNed 1 ==
  data: posizione input; posizione_NED output
function posizione_NED = wgs84toNed(posizione)

coder.extrinsic('evalin', 'wgs84Ellipsoid', 'geodetic2ned');
NED_origin = [0;0;0];
posizione_NED  = [0;0;0];
NED_origin = evalin('base', 'NED_origin');
[a, b, c] = geodetic2ned(posizione(1), posizione(2), posizione(3), NED_origin(1), NED_origin(2), NED_origin(3), wgs84Ellipsoid);
posizione_NED = [a; b; posizione(3)];

end

== matlab function TeamA_PAsqualo1/Navigazione/Correzione/MATLAB Function ==
  settings: updateMethod=DISCRETE
  data: col output size=[1 5]; u input; row output size=[1 5]; run output
function [col ,row, run] = select(u)

    run = 0;
    row = [];
    col = [];
    
    if u(1) == 1 % gps
        row = [row 1 2];
        col = [col 1 2];
        run = 1;
    end
    if u(2) == 1 % usbl
        row = [row 3 4];
        col = [col 3 4];
        run = 1;
    end
    if u(3) == 1 % depth
        row = [row 5];
        col = [col 5];
        run = 1;
    end

   
end

== matlab function TeamA_PAsqualo1/Navigazione/Correzione/MATLAB Function1 ==
  data: y_true input size=[n_meas_filter 1]; e output size=[n_meas_filter 1]; y_virt input size=[n_meas_filter 1]; select input
function e = innov_calc(y_true, y_virt, select)
% innov calc

e = y_true - y_virt;

% se e` pronta la misura dell'usbl,  calcolo
if select(2) == 1
	index = 2*select(1)+1;
	e(index,1) = atan2(sin(e(index,1)), cos(e(index,1)));
end


end

== matlab function TeamA_PAsqualo1/Navigazione/Correzione/kalman correction ==
  data: x_old input; x_new output size=[3 1]; P_old input; e input size=[n_meas_filter 1]; P_new output; S input size=[n_meas_filter n_meas_filter]; C input size=[n_state_filter n_meas_filter]
function [x_new, P_new]= kalman_correction(x_old, P_old, e, S, C)

	K = C*(S^-1); 
    P_delta = - K*S*K';
	
    x_new = x_old + K*e;
    P = P_old + P_delta;    
	
	P_new = (P+P')/2;
end
